simulink model "excs6_7"  (R2021a)
settings: Solver=FixedStepDiscrete  StartTime=0.0  StopTime=40  RelTol=1e-3
values from neighbouring files (symbols this model uses):
  A = [1 0; -1 0; 0 1; 0 -1]    [exc6.m]    (also in exc6_continue.m = [1 1; 0 1])
  B = [0; 1]    [exc6_continue.m]
  x0 = [10; 0]    [exc6_continue.m]
libraries: simulink x1
settings Model: Creator=emily  LastModifiedBy=davidrico

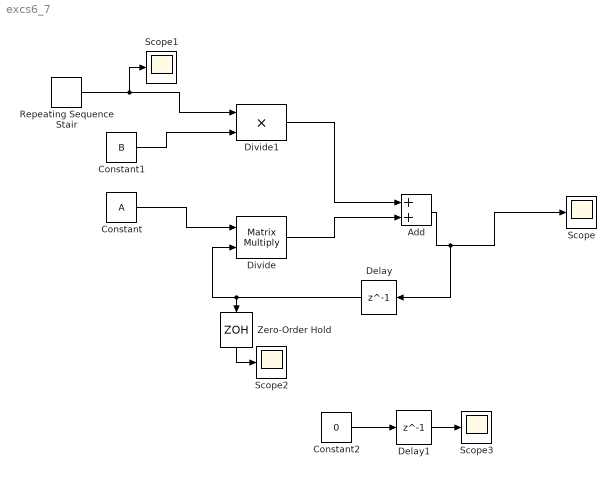
== system excs6_7 ==
  Add : Sum
  Constant : Constant  Value=A
  Constant1 : Constant  Value=B
  Constant2 : Constant  Value=0
  Delay : Delay  DelayLength=1  InitialCondition=x0  SampleTime=1
  Delay1 : Delay  DelayLength=1  InitialCondition=x0  SampleTime=1
  Divide : Product  Inputs=**  Multiplication=Matrix(*)
  Divide1 : Product  Inputs=**
  Repeating Sequence Stair : simulink/Sources/Repeating Sequence Stair  OutValues=u_res  tsamp=1  OutMin=[]  OutMax=[]  OutDataTypeStr=double  OutputDataTypeScalingMode=double  OutDataType=fixdt(0,8)  ConRadixGroup=Best Precision: Vector-wise  OutScaling=2^-12
  Scope{,1..3} (4 alike) : Scope
  Zero-Order Hold : ZeroOrderHold
  wires:
  Divide/1 -> Add/2
  Add/1 -> Delay/1, Scope/1
  Divide1/1 -> Add/1
  Constant1/1 -> Divide1/2
  Constant/1 -> Divide/1
  Repeating Sequence Stair/1 -> Scope1/1, Divide1/1
  Delay/1 -> Divide/2, Zero-Order Hold/1
  Zero-Order Hold/1 -> Scope2/1
  Delay1/1 -> Scope3/1
  Constant2/1 -> Delay1/1
